simulink model "F_control_system_sim"  (R2015a)
settings: Solver=ode45  SolverMode=SingleTasking  StartTime=0.0  StopTime=5  RelTol=1e-3
InitFcn:
  | ImportVars
undefined symbols (not defined in the file or in its folder): Kp, Kv
settings Model: CovMetricSettings=dwe  CovHtmlReporting=off  covSaveCumulativeToWorkspaceVar=off  CovSaveSingleToWorkspaceVar=off  CovExternalEMLEnable=on  Creator=soren  LastModifiedBy=JayJay
settings DataIOCC: LimitDataPoints=off  SaveFormat=Dataset
settings DebuggingCC: SFUnexpectedBacktrackingDiag=error  SFNoUnconditionalDefaultTransitionDiag=error
settings HardwareCC: ProdBitPerPointer=64  ProdLargestAtomicFloat=Float  ProdIntDivRoundTo=Zero  ProdEndianess=LittleEndian  ProdHWDeviceType=Specified
settings ModelReferenceCC: PropagateSignalLabelsOutOfModel=on
settings GRTTargetCC: TargetLangStandard=C99 (ISO)  GeneratePreprocessorConditionals=Use local settings

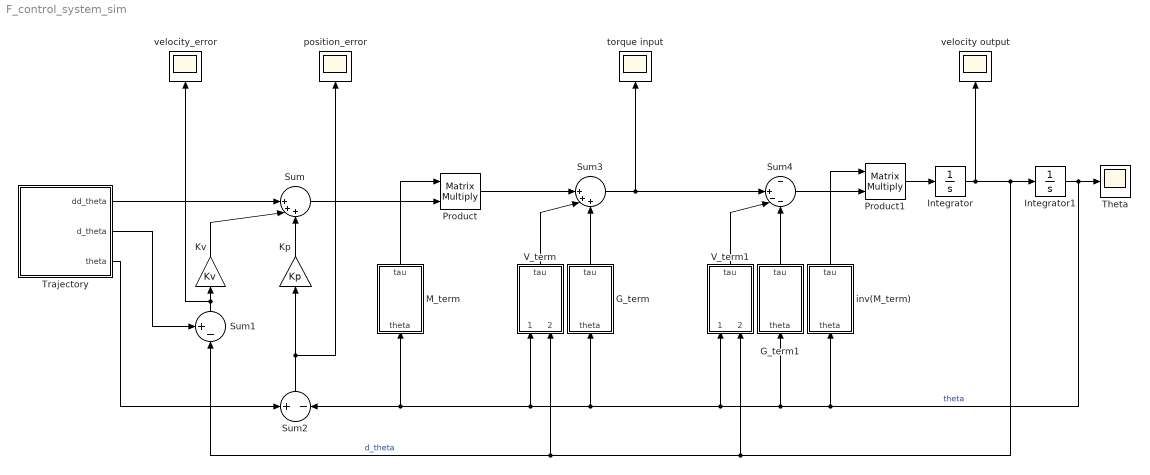
== system F_control_system_sim ==
  " G_term1" : Subsystem
  G_term : Subsystem
  Integrator : Integrator
  Integrator1 : Integrator  InitialCondition=[0; pi/2; 0]
  Kp : Gain  Gain=Kp
  Kv : Gain  Gain=Kv
  M_term : Subsystem
  Product : Product  Multiplication=Matrix(*)
  Product1 : Product  Multiplication=Matrix(*)
  Sum : Sum  Inputs=||+++
  Sum1 : Sum  Inputs=+-|
  Sum2 : Sum  Inputs=+|-
  Sum3 : Sum  Inputs=||+++
  Sum4 : Sum  Inputs=-|+--
  Theta : Scope
      settings: TimeRange=auto  ShowLegends=on  MaxDataPoints=5000  SaveToWorkspace=off  SaveName=ScopeData  YMin=-0.32135  YMax=2.89215  SampleTime=-1
  Trajectory : Subsystem
  V_term : Subsystem
  V_term1 : Subsystem
  inv(M_term) : Subsystem
  position_error : Scope
      settings: TimeRange=auto  ShowLegends=on  MaxDataPoints=5000  SaveToWorkspace=off  SaveName=ScopeData3  YMin=-0.125  YMax=1.125  SampleTime=-1
  torque input : Scope
      settings: TimeRange=auto  MaxDataPoints=5000  SaveToWorkspace=off  YMin=-10  YMax=10  SampleTime=-1
  velocity output : Scope
      settings: TimeRange=auto  ShowLegends=on  MaxDataPoints=5000  SaveToWorkspace=off  YMin=-0.14893  YMax=1.3404  SampleTime=-1
  velocity_error : Scope
      settings: TimeRange=auto  ShowLegends=on  MaxDataPoints=5000  SaveToWorkspace=off  SaveName=ScopeData2  YMin=-1.3404  YMax=0.14893  SampleTime=-1
  wires:
  Trajectory/2(d_theta) -> Sum1/1
  Trajectory/3(theta) -> Sum2/1
  Sum1/1 -> velocity_error/1, Kv/1
  Kv/1 -> Sum/2
  Sum2/1 -> Kp/1, position_error/1
  Kp/1 -> Sum/3
  Integrator/1 -> Integrator1/1, Sum1/2, V_term/2(d_theta), V_term1/2(d_theta), velocity output/1  "d_theta"
  Sum/1 -> Product/2
  Integrator1/1 -> Sum2/2, M_term/1(theta), V_term/1(theta), G_term/1(theta), V_term1/1(theta), " G_term1"/1(theta), inv(M_term)/1(theta), Theta/1  "theta"
  M_term/1(tau) -> Product/1
  Product/1 -> Sum3/1
  G_term/1(tau) -> Sum3/3
  V_term/1(tau) -> Sum3/2
  V_term1/1(tau) -> Sum4/3
  " G_term1"/1(tau) -> Sum4/4
  inv(M_term)/1(tau) -> Product1/1
  Sum3/1 -> torque input/1, Sum4/2
  Trajectory/1(dd_theta) -> Sum/1
  Sum4/1 -> Product1/2
  Product1/1 -> Integrator/1

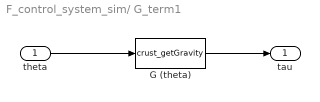
== system F_control_system_sim/ G_term1 ==
  theta : Inport
  G (theta) : MATLABFcn  MATLABFcn=crust_getGravity  OutputDimensions=[3 1]  OutputSignalType=real  Output1D=off
  tau : Outport
  wires:
  G (theta)/1 -> tau/1
  theta/1 -> G (theta)/1

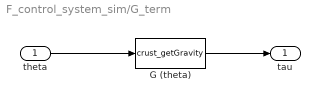
== system F_control_system_sim/G_term ==
  theta : Inport
  G (theta) : MATLABFcn  MATLABFcn=crust_getGravity  OutputDimensions=[3 1]  OutputSignalType=real  Output1D=off
  tau : Outport
  wires:
  G (theta)/1 -> tau/1
  theta/1 -> G (theta)/1

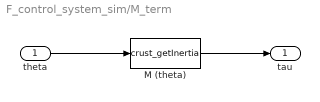
== system F_control_system_sim/M_term ==
  theta : Inport
  M (theta) : MATLABFcn  MATLABFcn=crust_getInertia  OutputDimensions=[3 3]  OutputSignalType=real  Output1D=off
  tau : Outport
  wires:
  theta/1 -> M (theta)/1
  M (theta)/1 -> tau/1

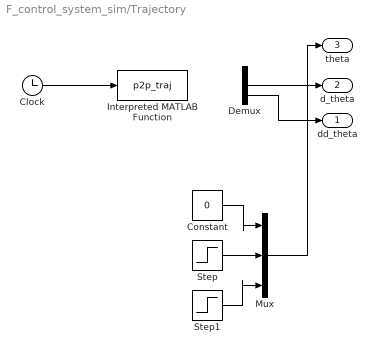
== system F_control_system_sim/Trajectory ==
  Clock : Clock
  Constant : Constant  Value=0
  Demux : Demux  Outputs=3
  Interpreted MATLAB Function : MATLABFcn  MATLABFcn=p2p_traj  OutputDimensions=9  OutputSignalType=real  Output1D=off
  Mux : Mux  Inputs=3
  Step : Step  Time=0  Before=pi/2  After=pi/2+1  SampleTime=0
  Step1 : Step  Time=0  SampleTime=0
  dd_theta : Outport
  d_theta : Outport  Port=2
  theta : Outport  Port=3
  wires:
  Clock/1 -> Interpreted MATLAB Function/1
  Demux/2 -> d_theta/1
  Demux/3 -> dd_theta/1
  Step/1 -> Mux/2
  Constant/1 -> Mux/1
  Step1/1 -> Mux/3
  Mux/1 -> theta/1

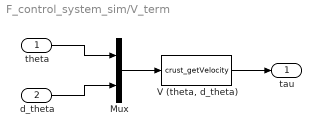
== system F_control_system_sim/V_term ==
  theta : Inport
  d_theta : Inport  Port=2
  Mux : Mux  Inputs=2
  "V (theta, d_theta)" : MATLABFcn  MATLABFcn=crust_getVelocity  OutputDimensions=[3 1]  OutputSignalType=real  Output1D=off
  tau : Outport
  wires:
  "V (theta, d_theta)"/1 -> tau/1
  theta/1 -> Mux/1
  d_theta/1 -> Mux/2
  Mux/1 -> "V (theta, d_theta)"/1

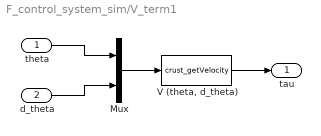
== system F_control_system_sim/V_term1 ==
  theta : Inport
  d_theta : Inport  Port=2
  Mux : Mux  Inputs=2
  "V (theta, d_theta)" : MATLABFcn  MATLABFcn=crust_getVelocity  OutputDimensions=[3 1]  OutputSignalType=real  Output1D=off
  tau : Outport
  wires:
  "V (theta, d_theta)"/1 -> tau/1
  theta/1 -> Mux/1
  d_theta/1 -> Mux/2
  Mux/1 -> "V (theta, d_theta)"/1

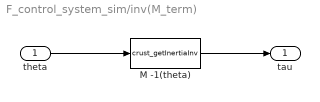
== system F_control_system_sim/inv(M_term) ==
  theta : Inport
  M -1(theta) : MATLABFcn  MATLABFcn=crust_getInertiaInv  OutputDimensions=[3 3]  OutputSignalType=real  Output1D=off
  tau : Outport
  wires:
  theta/1 -> M -1(theta)/1
  M -1(theta)/1 -> tau/1
